simulink model "hw6"  (R2019a)
settings: Solver=VariableStepAuto  StartTime=0.0  StopTime=150  RelTol=1e-3
settings Model: Creator=sumli  LastModifiedBy=sumli

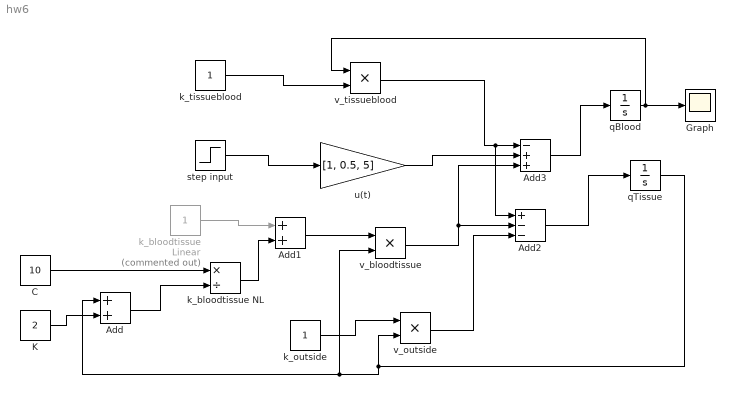
== system hw6 ==
  Add : Sum
  Add1 : Sum
  Add2 : Sum  Inputs=+--
  Add3 : Sum  Inputs=-++
  C : Constant  Value=10
  Graph : Scope
  K : Constant  Value=2
  k_bloodtissue Linear : Constant  Commented=on
  "k_bloodtissue NL " : Product  Inputs=*/
  k_outside : Constant
  k_tissueblood : Constant
  qBlood : Integrator
  qTissue : Integrator
  step input : Step  SampleTime=0
  u(t) : Gain  Gain=[1, 0.5, 5]
  v_bloodtissue : Product
  v_outside : Product
  v_tissueblood : Product
  wires:
  K/1 -> Add/2
  C/1 -> "k_bloodtissue NL "/1
  Add/1 -> "k_bloodtissue NL "/2
  step input/1 -> u(t)/1
  k_tissueblood/1 -> v_tissueblood/2
  qBlood/1 -> v_tissueblood/1, Graph/1
  k_bloodtissue Linear/1 -> Add1/1
  "k_bloodtissue NL "/1 -> Add1/2
  Add1/1 -> v_bloodtissue/1
  k_outside/1 -> v_outside/1
  u(t)/1 -> Add3/2
  Add2/1 -> qTissue/1
  Add3/1 -> qBlood/1
  qTissue/1 -> v_outside/2, Add/1, v_bloodtissue/2
  v_outside/1 -> Add2/3
  v_bloodtissue/1 -> Add3/3, Add2/2
  v_tissueblood/1 -> Add2/1, Add3/1
